simulink model "master_task"  (Simulink 3.0)
libraries: mathlib x8, inoutlib x1

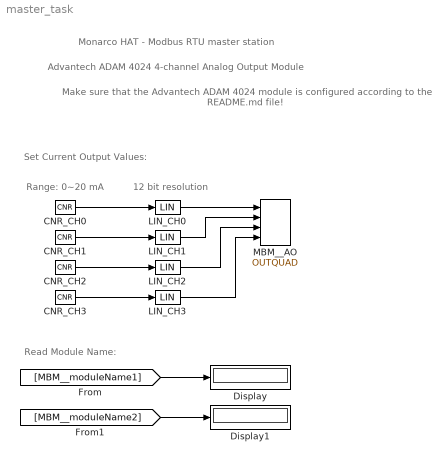
== system master_task ==
  note: Read Module Name:
  note: 12 bit resolution
  note: Range: 0~20 mA
  note: Advantech ADAM 4024 4-channel Analog Output Module
  note: Set Current Output Values:
  note: Make sure that the Advantech ADAM 4024 module is configured according to the README.md file!
  note: Monarco HAT - Modbus RTU master station
  CNR_CH{0..3} (4 alike) : mathlib/CNR  ycn=0
  Display : Display
      settings: Format=hex
  Display1 : Display
      settings: Format=hex
  LIN_CH{0..3} (4 alike) : mathlib/LIN  u1=0  y1=0  u2=20  y2=4095
  MBM__AO : inoutlib/OUTQUAD
  wires:
  CNR_CH0/1 -> LIN_CH0/1
  CNR_CH1/1 -> LIN_CH1/1
  CNR_CH2/1 -> LIN_CH2/1
  CNR_CH3/1 -> LIN_CH3/1
  [MBM__moduleName1] -> Display/1
  [MBM__moduleName2] -> Display1/1
  LIN_CH0/1 -> MBM__AO/1
  LIN_CH1/1 -> MBM__AO/2
  LIN_CH2/1 -> MBM__AO/3
  LIN_CH3/1 -> MBM__AO/4
